simulink model "Tarea1"  (R2025a)
settings: Solver=VariableStepAuto  StartTime=0.0  StopTime=10  RelTol=1e-3
values from neighbouring files (symbols this model uses):
  beq = 4.3    [matlab.mat]
  bp = 0.0024    [matlab.mat]
  fc = 0    [matlab.mat]
  g = 9.81    [matlab.mat]
  ip = 0.0079    [matlab.mat]
  lp = 0.3302    [matlab.mat]
  mc = 0.7031    [matlab.mat]
  mp = 0.23    [matlab.mat]
settings Model: Creator=carlo  LastModifiedBy=carlo

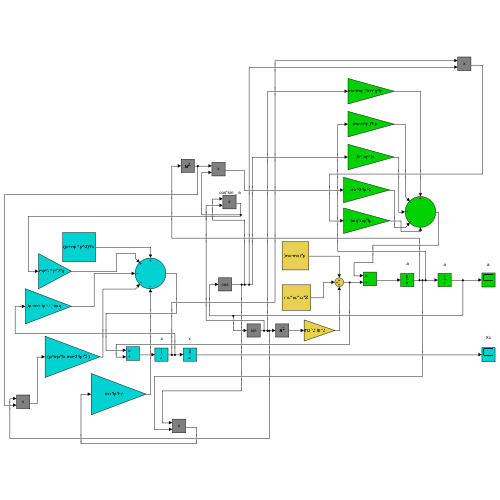
[thumbnail: Simulink's stored preview of the top-level diagram]
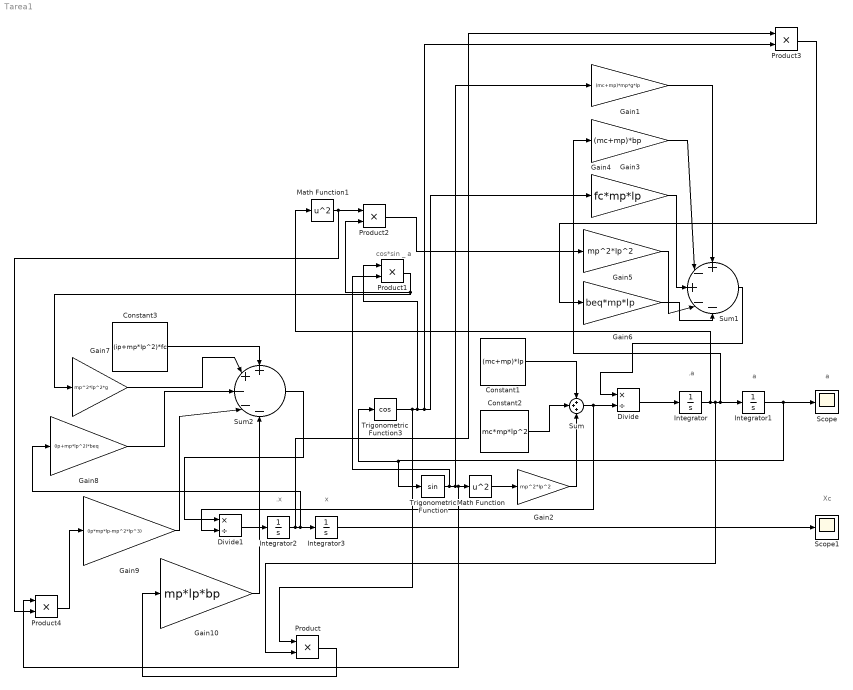
== system Tarea1 ==
  note: a
  note: Xc
  note: cos*sin _ a
  note: x
  note: .x
  note: a
  note: .a
  Constant1 : Constant  Value=(mc+mp)*lp
  Constant2 : Constant  Value=mc*mp*lp^2
  Constant3 : Constant  Value=(ip+mp*lp^2)*fc
  Divide : Product  Inputs=*/
  Divide1 : Product  Inputs=*/
  Gain1 : Gain  Gain=(mc+mp)*mp*g*lp
  Gain10 : Gain  Gain=mp*lp*bp
  Gain2 : Gain  Gain=mp^2*lp^2
  Gain3 : Gain  Gain=(mc+mp)*bp
  Gain4 : Gain  Gain=fc*mp*lp
  Gain5 : Gain  Gain=mp^2*lp^2
  Gain6 : Gain  Gain=beq*mp*lp
  Gain7 : Gain  Gain=mp^2*lp^2*g
  Gain8 : Gain  Gain=(ip+mp*lp^2)*beq
  Gain9 : Gain  Gain=(ip*mp*lp-mp^2*lp^3)
  Integrator : Integrator
  Integrator1 : Integrator  InitialCondition=1
  Integrator2 : Integrator
  Integrator3 : Integrator
  Math Function : Math  Operator=square
  Math Function1 : Math  Operator=square
  Product{,1..4} (5 alike) : Product
  Scope : Scope
      settings: ActiveDisplayYMinimum=0.46780138436015184  ActiveDisplayYMaximum=5.7897875407586348
  Scope1 : Scope
      settings: ActiveDisplayYMinimum=-0.13915027667620616  ActiveDisplayYMaximum=0.094984177857200425
  Sum : Sum  Inputs=+++
  Sum1 : Sum  Inputs=+-+--
  Sum2 : Sum  Inputs=++---
  Trigonometric Function : Trigonometry
  Trigonometric Function3 : Trigonometry  Operator=cos
  wires:
  Constant1/1 -> Sum/1
  Trigonometric Function/1 -> Product1/2, Gain1/1, Product4/1, Math Function/1
  Constant2/1 -> Sum/2
  Math Function/1 -> Gain2/1
  Gain2/1 -> Sum/3
  Divide/1 -> Integrator/1
  Integrator1/1 -> Trigonometric Function3/1, Trigonometric Function/1, Scope/1
  Sum1/1 -> Divide/1
  Gain1/1 -> Sum1/1
  Gain3/1 -> Sum1/2
  Gain4/1 -> Sum1/3
  Trigonometric Function3/1 -> Product/1, Product1/1, Product3/2, Gain4/1
  Gain5/1 -> Sum1/4
  Product1/1 -> Gain7/1, Product2/2
  Math Function1/1 -> Product4/2, Product2/1
  Product2/1 -> Gain5/1
  Product3/1 -> Gain6/1
  Gain6/1 -> Sum1/5
  Divide1/1 -> Integrator2/1
  Integrator2/1 -> Product3/1, Gain8/1, Integrator3/1
  Integrator3/1 -> Scope1/1
  Sum/1 -> Divide1/2, Divide/2
  Constant3/1 -> Sum2/1
  Gain7/1 -> Sum2/2
  Sum2/1 -> Divide1/1
  Gain8/1 -> Sum2/3
  Gain9/1 -> Sum2/4
  Integrator/1 -> Math Function1/1, Product/2, Gain3/1, Integrator1/1
  Product/1 -> Gain10/1
  Gain10/1 -> Sum2/5
  Product4/1 -> Gain9/1
